simulink model "INS"  (R2018b)
settings: configuration reference "ins_config" (kept outside this file)
undefined symbols (not defined in the file): DiscIntNeverNeededParam, INS_CONST, INS_EXPORT, INS_EXPORT_VALUE, INS_PARAM, Sensor_Meas
libraries: simulink x155, FMT_Model_Lib x52
(part 5 of 6)

== system INS/Data_Fusion/Translation_Filter/TF_Data_PreProcess/Sensor_Process/TF_Sensor_Measures/ExternalPos_Meas/External_Pos_PreProcess ==
  Sensor_Data : Inport
  Rotation_Data : Inport  Port=2
  Bus Selector2 : BusSelector  OutputSignals=ExternalPos_Data.x,ExternalPos_Data.y,ExternalPos_Data.h
  Bus Selector5 : BusSelector  OutputSignals=ExternalPos_Data.timestamp
  Demux : Demux  Outputs=3
  Local_To_Global : Subsystem
  Multiply : Product  Multiplication=Matrix(*)
  Mux : Mux  Inputs=3
  Reshape : Reshape  OutputDimensionality=Column vector (2-D)
  timestamp : Outport  VectorParamsAs1DForOutWhenUnconnected=off
  x : Outport  Port=2  VectorParamsAs1DForOutWhenUnconnected=off
  y : Outport  Port=3  VectorParamsAs1DForOutWhenUnconnected=off
  h : Outport  Port=4  VectorParamsAs1DForOutWhenUnconnected=off
  wires:
  Bus Selector2/2 -> Mux/2  "<y>"
  Mux/1 -> Reshape/1  "xyh_local"
  Multiply/1 -> Demux/1
  Demux/1 -> x/1
  Demux/2 -> y/1
  Bus Selector2/3 -> Mux/3  "<h>"
  Reshape/1 -> Multiply/2
  Bus Selector2/1 -> Mux/1  "<x>"
  Demux/3 -> h/1
  Bus Selector5/1 -> timestamp/1  "<timestamp>"
  Sensor_Data/1 -> Bus Selector5/1, Local_To_Global/1(Sensor_Data), Bus Selector2/1
  Rotation_Data/1 -> Local_To_Global/2(Rotation_Data)
  Local_To_Global/1(M_OC) -> Multiply/1

== system INS/Data_Fusion/Translation_Filter/TF_Data_PreProcess/TF_Data_Post_Process/GPS_OFFSET_Compensation/GPS_POS_Compensation/WGS_To_Global ==
  TF_Data : Inport
  Bus Selector : BusSelector  OutputSignals=Sensor_Meas.GPS_Meas.lat_rad,Sensor_Meas.GPS_Meas.lon_rad,Sensor_Meas.GPS_Meas.h_m,TF_Control.WGS84_Ref.WGS84_pos_ref.lat_0_rad,TF_Control.WGS84_Ref.WGS84_pos_ref.lon_0_rad,TF_Control.WGS84_Ref.WGS84_pos_ref.h_0_m,TF_Control.WGS84_Ref.WGS84_derivatives_ref.dx_dlat_0,TF_Control.WGS84_Ref.WGS84_derivatives_ref.dy_dlon_0,TF_Control.WGS84_Ref.WGS84_derivatives_ref.dz_dh_0
  Multiply : Product
  Mux : Mux  Inputs=3
  Mux1 : Mux  Inputs=3
  Mux2 : Mux  Inputs=3
  Sum : Sum  Inputs=|+-
  pos_O_m : Outport  VectorParamsAs1DForOutWhenUnconnected=off
  wires:
  Bus Selector/2 -> Mux/2  "<lon_rad>"
  Bus Selector/6 -> Mux1/3  "<h_0_m>"
  Bus Selector/3 -> Mux/3  "<h_m>"
  Mux1/1 -> Sum/2
  Bus Selector/4 -> Mux1/1  "<lat_0_rad>"
  Sum/1 -> Multiply/1
  Mux2/1 -> Multiply/2
  Bus Selector/1 -> Mux/1  "<lat_rad>"
  Bus Selector/5 -> Mux1/2  "<lon_0_rad>"
  Mux/1 -> Sum/1
  TF_Data/1 -> Bus Selector/1
  Multiply/1 -> pos_O_m/1
  Bus Selector/7 -> Mux2/1  "<dx_dlat_0>"
  Bus Selector/8 -> Mux2/2  "<dy_dlon_0>"
  Bus Selector/9 -> Mux2/3  "<dz_dh_0>"

== system INS/Data_Fusion/Translation_Filter/TF_Data_PreProcess/TF_Data_Post_Process/GPS_OFFSET_Compensation/GPS_VEL_Compensation/delay ==
  u : Inport
  Divide : Product  Inputs=*/
  Mux : Mux  Inputs=3
  Selector : Selector  InputPortWidth=3  IndexOptions=Index vector (dialog)  Indices=1  OutputSizes=1
  Selector1 : Selector  InputPortWidth=3  IndexOptions=Index vector (dialog)  Indices=2  OutputSizes=1
  Selector2 : Selector  InputPortWidth=3  IndexOptions=Index vector (dialog)  Indices=3  OutputSizes=1
  gps_vd_delay : Delay  DelayLengthSource=Input port  DelayLength=INS_PARAM.GPS_VEL_DELAY/INS_EXPORT.period  DelayLengthUpperLimit=500  InitialConditionSource=Input port
      settings: InputPortMap=u0,p1,p4
  gps_ve_delay : Delay  DelayLengthSource=Input port  DelayLength=INS_PARAM.GPS_VEL_DELAY/INS_EXPORT.period  DelayLengthUpperLimit=500  InitialConditionSource=Input port
      settings: InputPortMap=u0,p1,p4
  gps_vnl_delay : Delay  DelayLengthSource=Input port  DelayLength=INS_PARAM.GPS_VEL_DELAY/INS_EXPORT.period  DelayLengthUpperLimit=500  InitialConditionSource=Input port
      settings: InputPortMap=u0,p1,p4
  period : Constant  Value=INS_EXPORT.period
  vel_delay : Constant  Value=INS_PARAM.GPS_VEL_DELAY
  y : Outport  VectorParamsAs1DForOutWhenUnconnected=off
  wires:
  u/1 -> Selector2/1, Selector1/1, Selector/1
  Divide/1 -> gps_vnl_delay/2, gps_vd_delay/2, gps_ve_delay/2
  vel_delay/1 -> Divide/1
  Selector/1 -> gps_vnl_delay/3, gps_vnl_delay/1
  Selector1/1 -> gps_ve_delay/3, gps_ve_delay/1
  Selector2/1 -> gps_vd_delay/3, gps_vd_delay/1
  gps_vnl_delay/1 -> Mux/1
  gps_ve_delay/1 -> Mux/2
  gps_vd_delay/1 -> Mux/3
  Mux/1 -> y/1
  period/1 -> Divide/2

== system INS/Data_Fusion/Translation_Filter/TF_Data_PreProcess/Transfer_Filter_Control/Sensor_Valid/Horizon_Sensor_Valid/valid_hold ==
  u : Inport
  Compare To Constant : simulink/Logic and Bit Operations/Compare To Constant  relop=>=  const=time_out  OutDataTypeStr=boolean
  Compare To Constant1 : simulink/Logic and Bit Operations/Compare To Constant  relop=>  const=0  OutDataTypeStr=boolean
  Compare To Constant2 : simulink/Logic and Bit Operations/Compare To Constant  relop=>  const=0  OutDataTypeStr=boolean
  Constant : Constant  Value=INS_EXPORT.period  OutDataTypeStr=uint32
  Delay : Delay  DelayLength=1
  Detect Rise Positive : simulink/Logic and Bit Operations/Detect Rise Positive  vinit=0  OutDataTypeStr=boolean
  Discrete-Time Integrator : DiscreteIntegrator  IntegratorMethod=Accumulation: Forward Euler  gainval=1  ExternalReset=level  SampleTime=-1  LimitOutput=on  UpperSaturationLimit=1e6  LowerSaturationLimit=0  ICPrevOutput=DiscIntNeverNeededParam  ICPrevScaledInput=DiscIntNeverNeededParam
  Logical Operator : Logic  Operator=NOT  AllPortsSameDT=off  OutDataTypeStr=boolean
  Logical Operator1 : Logic  Operator=OR  AllPortsSameDT=off  OutDataTypeStr=boolean
  Multiply : Product
  y : Outport  VectorParamsAs1DForOutWhenUnconnected=off
  wires:
  Multiply/1 -> y/1
  Logical Operator1/1 -> Multiply/2, Delay/1
  Detect Rise Positive/1 -> Logical Operator1/1
  Compare To Constant2/1 -> Detect Rise Positive/1
  u/1 -> Compare To Constant1/1, Compare To Constant2/1
  Compare To Constant1/1 -> Discrete-Time Integrator/2
  Constant/1 -> Discrete-Time Integrator/1
  Compare To Constant/1 -> Logical Operator/1
  Logical Operator/1 -> Multiply/1
  Discrete-Time Integrator/1 -> Compare To Constant/1
  Delay/1 -> Logical Operator1/2

== system INS/Data_Fusion/Translation_Filter/TF_Data_PreProcess/Transfer_Filter_Control/Sensor_Valid/Horizon_Sensor_Valid/valid_hold1 ==
  u : Inport
  Compare To Constant : simulink/Logic and Bit Operations/Compare To Constant  relop=>=  const=time_out  OutDataTypeStr=boolean
  Compare To Constant1 : simulink/Logic and Bit Operations/Compare To Constant  relop=>  const=0  OutDataTypeStr=boolean
  Compare To Constant2 : simulink/Logic and Bit Operations/Compare To Constant  relop=>  const=0  OutDataTypeStr=boolean
  Constant : Constant  Value=INS_EXPORT.period  OutDataTypeStr=uint32
  Delay : Delay  DelayLength=1
  Detect Rise Positive : simulink/Logic and Bit Operations/Detect Rise Positive  vinit=0  OutDataTypeStr=boolean
  Discrete-Time Integrator : DiscreteIntegrator  IntegratorMethod=Accumulation: Forward Euler  gainval=1  ExternalReset=level  SampleTime=-1  LimitOutput=on  UpperSaturationLimit=1e6  LowerSaturationLimit=0  ICPrevOutput=DiscIntNeverNeededParam  ICPrevScaledInput=DiscIntNeverNeededParam
  Logical Operator : Logic  Operator=NOT  AllPortsSameDT=off  OutDataTypeStr=boolean
  Logical Operator1 : Logic  Operator=OR  AllPortsSameDT=off  OutDataTypeStr=boolean
  Multiply : Product
  y : Outport  VectorParamsAs1DForOutWhenUnconnected=off
  wires:
  Discrete-Time Integrator/1 -> Compare To Constant/1
  Logical Operator/1 -> Multiply/1
  Compare To Constant/1 -> Logical Operator/1
  Constant/1 -> Discrete-Time Integrator/1
  Compare To Constant1/1 -> Discrete-Time Integrator/2
  u/1 -> Compare To Constant2/1, Compare To Constant1/1
  Compare To Constant2/1 -> Detect Rise Positive/1
  Detect Rise Positive/1 -> Logical Operator1/1
  Logical Operator1/1 -> Delay/1, Multiply/2
  Multiply/1 -> y/1
  Delay/1 -> Logical Operator1/2

== system INS/Data_Fusion/Translation_Filter/TF_Data_PreProcess/Transfer_Filter_Control/Sensor_Valid/Horizon_Sensor_Valid/valid_hold2 ==
  u : Inport
  Compare To Constant : simulink/Logic and Bit Operations/Compare To Constant  relop=>=  const=time_out  OutDataTypeStr=boolean
  Compare To Constant1 : simulink/Logic and Bit Operations/Compare To Constant  relop=>  const=0  OutDataTypeStr=boolean
  Compare To Constant2 : simulink/Logic and Bit Operations/Compare To Constant  relop=>  const=0  OutDataTypeStr=boolean
  Constant : Constant  Value=INS_EXPORT.period  OutDataTypeStr=uint32
  Delay : Delay  DelayLength=1
  Detect Rise Positive : simulink/Logic and Bit Operations/Detect Rise Positive  vinit=0  OutDataTypeStr=boolean
  Discrete-Time Integrator : DiscreteIntegrator  IntegratorMethod=Accumulation: Forward Euler  gainval=1  ExternalReset=level  SampleTime=-1  LimitOutput=on  UpperSaturationLimit=1e6  LowerSaturationLimit=0  ICPrevOutput=DiscIntNeverNeededParam  ICPrevScaledInput=DiscIntNeverNeededParam
  Logical Operator : Logic  Operator=NOT  AllPortsSameDT=off  OutDataTypeStr=boolean
  Logical Operator1 : Logic  Operator=OR  AllPortsSameDT=off  OutDataTypeStr=boolean
  Multiply : Product
  y : Outport  VectorParamsAs1DForOutWhenUnconnected=off
  wires:
  Delay/1 -> Logical Operator1/2
  Multiply/1 -> y/1
  Logical Operator1/1 -> Multiply/2, Delay/1
  Detect Rise Positive/1 -> Logical Operator1/1
  Compare To Constant2/1 -> Detect Rise Positive/1
  u/1 -> Compare To Constant1/1, Compare To Constant2/1
  Compare To Constant1/1 -> Discrete-Time Integrator/2
  Constant/1 -> Discrete-Time Integrator/1
  Compare To Constant/1 -> Logical Operator/1
  Logical Operator/1 -> Multiply/1
  Discrete-Time Integrator/1 -> Compare To Constant/1

== system INS/Data_Fusion/Translation_Filter/TF_Data_PreProcess/Transfer_Filter_Control/Sensor_Valid/Vertical_Sensor_Valid/valid_hold ==
  u : Inport
  Compare To Constant : simulink/Logic and Bit Operations/Compare To Constant  relop=>=  const=time_out  OutDataTypeStr=boolean
  Compare To Constant1 : simulink/Logic and Bit Operations/Compare To Constant  relop=>  const=0  OutDataTypeStr=boolean
  Compare To Constant2 : simulink/Logic and Bit Operations/Compare To Constant  relop=>  const=0  OutDataTypeStr=boolean
  Constant : Constant  Value=INS_EXPORT.period  OutDataTypeStr=uint32
  Delay : Delay  DelayLength=1
  Detect Rise Positive : simulink/Logic and Bit Operations/Detect Rise Positive  vinit=0  OutDataTypeStr=boolean
  Discrete-Time Integrator : DiscreteIntegrator  IntegratorMethod=Accumulation: Forward Euler  gainval=1  ExternalReset=level  SampleTime=-1  LimitOutput=on  UpperSaturationLimit=1e6  LowerSaturationLimit=0  ICPrevOutput=DiscIntNeverNeededParam  ICPrevScaledInput=DiscIntNeverNeededParam
  Logical Operator : Logic  Operator=NOT  AllPortsSameDT=off  OutDataTypeStr=boolean
  Logical Operator1 : Logic  Operator=OR  AllPortsSameDT=off  OutDataTypeStr=boolean
  Multiply : Product
  y : Outport  VectorParamsAs1DForOutWhenUnconnected=off
  wires:
  Multiply/1 -> y/1
  Logical Operator1/1 -> Multiply/2, Delay/1
  Detect Rise Positive/1 -> Logical Operator1/1
  Compare To Constant2/1 -> Detect Rise Positive/1
  u/1 -> Compare To Constant1/1, Compare To Constant2/1
  Compare To Constant1/1 -> Discrete-Time Integrator/2
  Constant/1 -> Discrete-Time Integrator/1
  Compare To Constant/1 -> Logical Operator/1
  Logical Operator/1 -> Multiply/1
  Discrete-Time Integrator/1 -> Compare To Constant/1
  Delay/1 -> Logical Operator1/2

== system INS/Data_Fusion/Translation_Filter/TF_Data_PreProcess/Transfer_Filter_Control/Sensor_Valid/Vertical_Sensor_Valid/valid_hold1 ==
  u : Inport
  Compare To Constant : simulink/Logic and Bit Operations/Compare To Constant  relop=>=  const=time_out  OutDataTypeStr=boolean
  Compare To Constant1 : simulink/Logic and Bit Operations/Compare To Constant  relop=>  const=0  OutDataTypeStr=boolean
  Compare To Constant2 : simulink/Logic and Bit Operations/Compare To Constant  relop=>  const=0  OutDataTypeStr=boolean
  Constant : Constant  Value=INS_EXPORT.period  OutDataTypeStr=uint32
  Delay : Delay  DelayLength=1
  Detect Rise Positive : simulink/Logic and Bit Operations/Detect Rise Positive  vinit=0  OutDataTypeStr=boolean
  Discrete-Time Integrator : DiscreteIntegrator  IntegratorMethod=Accumulation: Forward Euler  gainval=1  ExternalReset=level  SampleTime=-1  LimitOutput=on  UpperSaturationLimit=1e6  LowerSaturationLimit=0  ICPrevOutput=DiscIntNeverNeededParam  ICPrevScaledInput=DiscIntNeverNeededParam
  Logical Operator : Logic  Operator=NOT  AllPortsSameDT=off  OutDataTypeStr=boolean
  Logical Operator1 : Logic  Operator=OR  AllPortsSameDT=off  OutDataTypeStr=boolean
  Multiply : Product
  y : Outport  VectorParamsAs1DForOutWhenUnconnected=off
  wires:
  Discrete-Time Integrator/1 -> Compare To Constant/1
  Logical Operator/1 -> Multiply/1
  Compare To Constant/1 -> Logical Operator/1
  Constant/1 -> Discrete-Time Integrator/1
  Compare To Constant1/1 -> Discrete-Time Integrator/2
  u/1 -> Compare To Constant2/1, Compare To Constant1/1
  Compare To Constant2/1 -> Detect Rise Positive/1
  Detect Rise Positive/1 -> Logical Operator1/1
  Logical Operator1/1 -> Delay/1, Multiply/2
  Multiply/1 -> y/1
  Delay/1 -> Logical Operator1/2

== system INS/Data_Fusion/Translation_Filter/TF_Data_PreProcess/Transfer_Filter_Control/Sensor_Valid/Vertical_Sensor_Valid/valid_hold2 ==
  u : Inport
  Compare To Constant : simulink/Logic and Bit Operations/Compare To Constant  relop=>=  const=time_out  OutDataTypeStr=boolean
  Compare To Constant1 : simulink/Logic and Bit Operations/Compare To Constant  relop=>  const=0  OutDataTypeStr=boolean
  Compare To Constant2 : simulink/Logic and Bit Operations/Compare To Constant  relop=>  const=0  OutDataTypeStr=boolean
  Constant : Constant  Value=INS_EXPORT.period  OutDataTypeStr=uint32
  Delay : Delay  DelayLength=1
  Detect Rise Positive : simulink/Logic and Bit Operations/Detect Rise Positive  vinit=0  OutDataTypeStr=boolean
  Discrete-Time Integrator : DiscreteIntegrator  IntegratorMethod=Accumulation: Forward Euler  gainval=1  ExternalReset=level  SampleTime=-1  LimitOutput=on  UpperSaturationLimit=1e6  LowerSaturationLimit=0  ICPrevOutput=DiscIntNeverNeededParam  ICPrevScaledInput=DiscIntNeverNeededParam
  Logical Operator : Logic  Operator=NOT  AllPortsSameDT=off  OutDataTypeStr=boolean
  Logical Operator1 : Logic  Operator=OR  AllPortsSameDT=off  OutDataTypeStr=boolean
  Multiply : Product
  y : Outport  VectorParamsAs1DForOutWhenUnconnected=off
  wires:
  Delay/1 -> Logical Operator1/2
  Multiply/1 -> y/1
  Logical Operator1/1 -> Multiply/2, Delay/1
  Detect Rise Positive/1 -> Logical Operator1/1
  Compare To Constant2/1 -> Detect Rise Positive/1
  u/1 -> Compare To Constant1/1, Compare To Constant2/1
  Compare To Constant1/1 -> Discrete-Time Integrator/2
  Constant/1 -> Discrete-Time Integrator/1
  Compare To Constant/1 -> Logical Operator/1
  Logical Operator/1 -> Multiply/1
  Discrete-Time Integrator/1 -> Compare To Constant/1

== system INS/Data_Fusion/Rotation_Filter/AHRS/Correct/Attitude_Correction/Attitude_Correct/Acc_Correct/Heading_Correct ==
  acc_est_O_mPs2 : Inport
  acc_meas_O_mPs2 : Inport  Port=2
  acc_meas_valid : Inport  Port=3
  Cross Product : FMT_Model_Lib/Math/Cross Product
      settings: SourceProductName=FMT Toolbox
  Dead Zone2 : DeadZone  LowerValue=-0.2  UpperValue=0.2  SaturateOnIntegerOverflow=on
  Demux : Demux  Outputs=3
  Demux1 : Demux  Outputs=3
  Gain : Gain  Gain=INS_PARAM.HEADING_GAIN  OutDataTypeStr=single
  Gain1 : Gain  Gain=0
  Gain2 : Gain  Gain=0
  Multiply : Product
  Mux1 : Mux  Inputs=3
  Mux2 : Mux  Inputs=3
  Saturation : Saturate
  heading_correct : Outport  VectorParamsAs1DForOutWhenUnconnected=off
  wires:
  Dead Zone2/1 -> Gain/1
  Saturation/1 -> Multiply/1
  Mux1/1 -> Cross Product/2
  Cross Product/1 -> Dead Zone2/1
  Demux/1 -> Mux1/1
  acc_meas_valid/1 -> Multiply/2
  Multiply/1 -> heading_correct/1
  Gain/1 -> Saturation/1
  acc_meas_O_mPs2/1 -> Demux/1
  Demux/2 -> Mux1/2
  Demux/3 -> Gain1/1
  Gain1/1 -> Mux1/3
  Demux1/2 -> Mux2/2
  Mux2/1 -> Cross Product/1
  Gain2/1 -> Mux2/3
  Demux1/1 -> Mux2/1
  Demux1/3 -> Gain2/1
  acc_est_O_mPs2/1 -> Demux1/1

== system INS/Data_Fusion/Rotation_Filter/AHRS/Correct/Attitude_Correction/Attitude_Correct/Acc_Correct/Verticle_Correct ==
  acc_est_O_mPs2 : Inport
  acc_meas_O_mPs2 : Inport  Port=2
  Cross Product : FMT_Model_Lib/Math/Cross Product
      settings: SourceProductName=FMT Toolbox
  Demux : Demux  Outputs=3
  Gain : Gain  Gain=INS_PARAM.ATT_GAIN
  Gain1 : Gain  Gain=INS_PARAM.ATT_GAIN
  Gain2 : Gain  Gain=0
  Mux : Mux  Inputs=3
  Saturation : Subsystem
  Vector Normalize : FMT_Model_Lib/Math/Vector Normalize
      settings: SourceProductName=FMT Toolbox
  Vector Normalize1 : FMT_Model_Lib/Math/Vector Normalize
      settings: SourceProductName=FMT Toolbox
  vert_correct : Outport  VectorParamsAs1DForOutWhenUnconnected=off
  wires:
  Saturation/1(y) -> Demux/1
  Cross Product/1 -> Saturation/1(u)
  Vector Normalize/1 -> Cross Product/1
  acc_meas_O_mPs2/1 -> Vector Normalize1/1
  Mux/1 -> vert_correct/1
  acc_est_O_mPs2/1 -> Vector Normalize/1
  Vector Normalize1/1 -> Cross Product/2
  Demux/1 -> Gain/1
  Demux/2 -> Gain1/1
  Demux/3 -> Gain2/1
  Gain/1 -> Mux/1
  Gain1/1 -> Mux/2
  Gain2/1 -> Mux/3

== system INS/Data_Fusion/Rotation_Filter/AHRS/Correct/Attitude_Correction/Attitude_Correct/Acc_Estimator/Estimate_Acc ==
  gps_meas_valid : Inport
  Sensor_Data : Inport  Port=2
  Rotation_Data : Inport  Port=3
  Bus Selector : BusSelector  OutputSignals=IMU_Data.acc_B_mPs2
  Bus Selector1 : BusSelector  OutputSignals=M_OB
  Constant : Constant  Value=200  OutDataTypeStr=uint32
  Delay : Delay  DelayLengthSource=Input port  DelayLengthUpperLimit=200
      settings: InputPortMap=u0,p1
  Divide : Product  Inputs=*/
  GPS_Delay : Constant  Value=INS_EXPORT.period  OutDataTypeStr=uint32
  Multiply : Product  Multiplication=Matrix(*)
  Multiply2 : Product  OutDataTypeStr=single
  Second Order LPF : FMT_Model_Lib/Filter/Second Order LPF  fc=10  zeta=0.707
      settings: SourceProductName=FMT Toolbox
  acc_est_O_mPs2 : Outport  VectorParamsAs1DForOutWhenUnconnected=off
  wires:
  Second Order LPF/1 -> Delay/1
  Multiply/1 -> Second Order LPF/1  "acc_O"
  Bus Selector/1 -> Multiply/2  "<acc_B_mPs2>"
  Bus Selector1/1 -> Multiply/1  "<M_OB>"
  Rotation_Data/1 -> Bus Selector1/1
  Sensor_Data/1 -> Bus Selector/1
  Delay/1 -> acc_est_O_mPs2/1
  Multiply2/1 -> Delay/2
  Divide/1 -> Multiply2/2
  gps_meas_valid/1 -> Multiply2/1
  GPS_Delay/1 -> Divide/2
  Constant/1 -> Divide/1

== system INS/Data_Fusion/Rotation_Filter/AHRS/Correct/Attitude_Correction/Attitude_Correct/Acc_Estimator/Measure_Acc ==
  Sensor_Data : Inport
  Bus_Selection : Subsystem
  Detect Increase : simulink/Logic and Bit Operations/Detect Increase  vinit=0.0  OutDataTypeStr=boolean
  GPS_Meas_Acc : Subsystem  mask{fc=10, zeta=1}
      mask prompts: fc "Cut-off frequency (Hz)"; zeta "Damping factor"
  Valid_Check : Subsystem
  gps_meas_valid : Outport  VectorParamsAs1DForOutWhenUnconnected=off
  gps_meas_acc : Outport  Port=2  VectorParamsAs1DForOutWhenUnconnected=off
  wires:
  Valid_Check/1(gps_meas_acc_valid) -> gps_meas_valid/1, GPS_Meas_Acc/Enable, Detect Increase/1
  Detect Increase/1 -> GPS_Meas_Acc/1(reset)
  GPS_Meas_Acc/1(gps_acc_O_mPs2) -> gps_meas_acc/1
  Bus_Selection/1(gps_vel_O_mPs) -> GPS_Meas_Acc/2(gps_vel_O_mPs)
  Sensor_Data/1 -> Bus_Selection/1(Sensor_Data), Valid_Check/1(Sensor_Data)

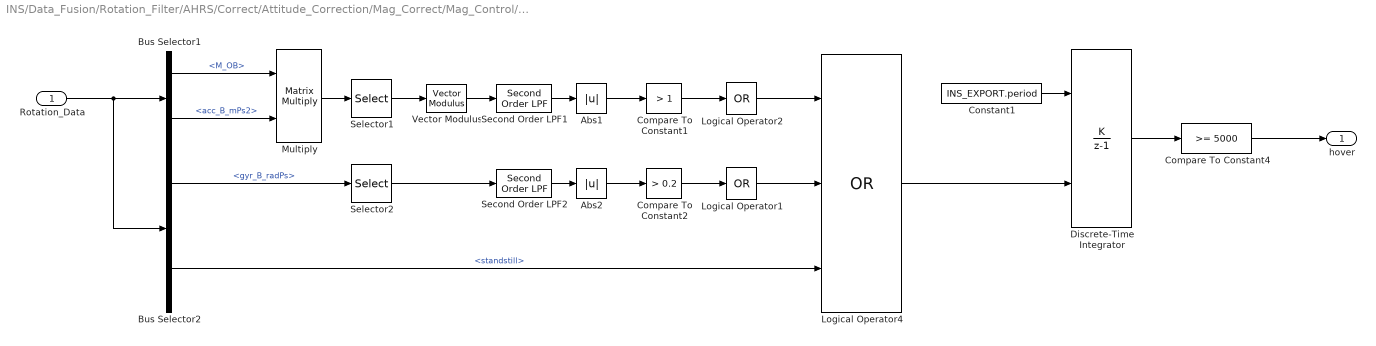
== system INS/Data_Fusion/Rotation_Filter/AHRS/Correct/Attitude_Correction/Mag_Correct/Mag_Control/Hover ==
  Rotation_Data : Inport
  Abs1 : Abs
  Abs2 : Abs
  Bus Selector1 : BusSelector  OutputSignals=M_OB,acc_B_mPs2
  Bus Selector2 : BusSelector  OutputSignals=gyr_B_radPs,standstill
  Compare To Constant1 : simulink/Logic and Bit Operations/Compare To Constant  relop=>  const=1  OutDataTypeStr=boolean
  Compare To Constant2 : simulink/Logic and Bit Operations/Compare To Constant  relop=>  const=0.2  OutDataTypeStr=boolean
  Compare To Constant4 : simulink/Logic and Bit Operations/Compare To Constant  relop=>=  const=5000  OutDataTypeStr=boolean
  Constant1 : Constant  Value=INS_EXPORT.period  OutDataTypeStr=uint32
  Discrete-Time Integrator : DiscreteIntegrator  IntegratorMethod=Accumulation: Forward Euler  ExternalReset=level  SampleTime=-1  OutDataTypeStr=uint32  SaturateOnIntegerOverflow=on  LimitOutput=on  UpperSaturationLimit=4294967295  LowerSaturationLimit=0  ICPrevOutput=DiscIntNeverNeededParam  ICPrevScaledInput=DiscIntNeverNeededParam
  Logical Operator1 : Logic  Operator=OR  Inputs=1  AllPortsSameDT=off  OutDataTypeStr=boolean
  Logical Operator2 : Logic  Operator=OR  Inputs=1  AllPortsSameDT=off  OutDataTypeStr=boolean
  Logical Operator4 : Logic  Operator=OR  Inputs=3  AllPortsSameDT=off  OutDataTypeStr=boolean
  Multiply : Product  Multiplication=Matrix(*)
  Second Order LPF1 : FMT_Model_Lib/Filter/Second Order LPF  fc=5  zeta=0.707
      settings: SourceProductName=FMT Toolbox
  Second Order LPF2 : FMT_Model_Lib/Filter/Second Order LPF  fc=5  zeta=0.707
      settings: SourceProductName=FMT Toolbox
  Selector1 : Selector  InputPortWidth=3  IndexOptions=Index vector (dialog)  Indices=[1 2]  OutputSizes=1
  Selector2 : Selector  InputPortWidth=3  IndexOptions=Index vector (dialog)  Indices=3  OutputSizes=1
  Vector Modulus : FMT_Model_Lib/Math/Vector Modulus
      settings: SourceProductName=FMT Toolbox
  hover : Outport  VectorParamsAs1DForOutWhenUnconnected=off
  wires:
  Discrete-Time Integrator/1 -> Compare To Constant4/1
  Logical Operator4/1 -> Discrete-Time Integrator/2
  Constant1/1 -> Discrete-Time Integrator/1
  Compare To Constant4/1 -> hover/1
  Rotation_Data/1 -> Bus Selector2/1, Bus Selector1/1
  Bus Selector1/2 -> Multiply/2  "<acc_B_mPs2>"
  Bus Selector1/1 -> Multiply/1  "<M_OB>"
  Multiply/1 -> Selector1/1
  Selector1/1 -> Vector Modulus/1
  Compare To Constant1/1 -> Logical Operator2/1
  Abs1/1 -> Compare To Constant1/1
  Logical Operator2/1 -> Logical Operator4/1
  Bus Selector2/1 -> Selector2/1  "<gyr_B_radPs>"
  Selector2/1 -> Second Order LPF2/1
  Second Order LPF2/1 -> Abs2/1
  Abs2/1 -> Compare To Constant2/1
  Compare To Constant2/1 -> Logical Operator1/1
  Logical Operator1/1 -> Logical Operator4/2
  Bus Selector2/2 -> Logical Operator4/3  "<standstill>"
  Second Order LPF1/1 -> Abs1/1
  Vector Modulus/1 -> Second Order LPF1/1

== system INS/Data_Fusion/Rotation_Filter/AHRS/Correct/Attitude_Correction/Mag_Correct/Mag_Measure/Bias_Estimation ==
  bias_update : Inport
  psi_meas : Inport  Port=2
  psi_est : Inport  Port=3
  standstill : Inport  Port=4
  Bias : Subsystem
  Delay : Delay  DelayLength=1
  Logical Operator1 : Logic  Operator=NOT  AllPortsSameDT=off  OutDataTypeStr=boolean
  Multiply : Product
  Switch : Switch  Criteria=u2 > Threshold  OutDataTypeStr=single
  bias : Outport  VectorParamsAs1DForOutWhenUnconnected=off
  wires:
  Delay/1 -> Switch/3
  Bias/1(bias) -> Switch/1
  Multiply/1 -> Delay/1, bias/1
  psi_meas/1 -> Bias/2(psi_meas)
  psi_est/1 -> Bias/1(psi_est)
  bias_update/1 -> Switch/2  "mag_bias_update"
  Switch/1 -> Multiply/2
  standstill/1 -> Logical Operator1/1
  Logical Operator1/1 -> Multiply/1

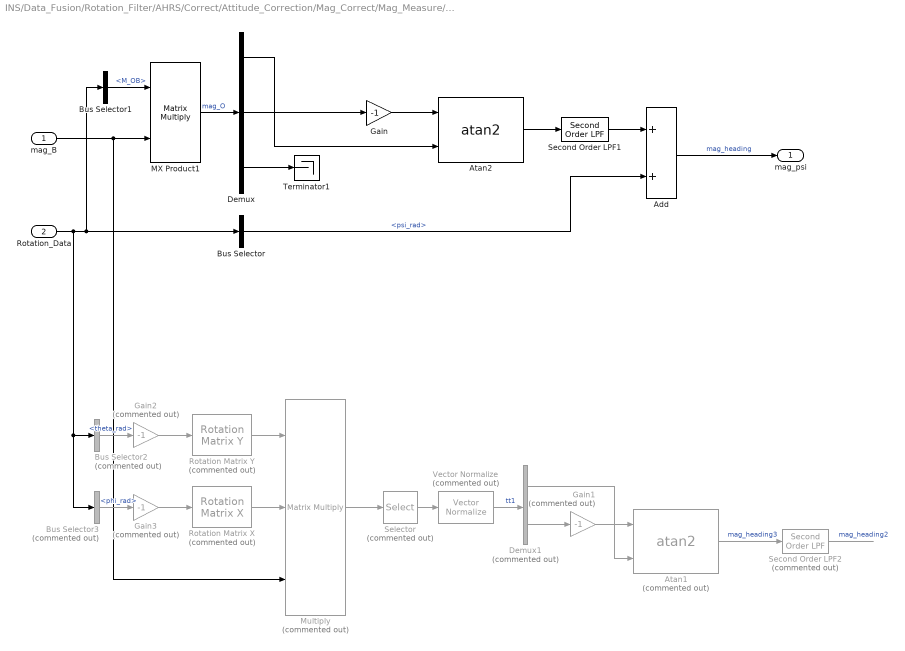
== system INS/Data_Fusion/Rotation_Filter/AHRS/Correct/Attitude_Correction/Mag_Correct/Mag_Measure/Mag_Heading ==
  mag_B : Inport
  Rotation_Data : Inport  Port=2
  Add : Sum
  Atan1 : Trigonometry  Commented=on  Operator=atan2
  Atan2 : Trigonometry  Operator=atan2
  Bus Selector : BusSelector  OutputSignals=psi_rad
  Bus Selector1 : BusSelector  OutputSignals=M_OB
  Bus Selector2 : BusSelector  Commented=on  OutputSignals=theta_rad
  Bus Selector3 : BusSelector  Commented=on  OutputSignals=phi_rad
  Demux : Demux  Outputs=3
  Demux1 : Demux  Commented=on  Outputs=2
  Gain : Gain  Gain=-1
  Gain1 : Gain  Commented=on  Gain=-1
  Gain2 : Gain  Commented=on  Gain=-1
  Gain3 : Gain  Commented=on  Gain=-1
  MX Product1 : Product  Multiplication=Matrix(*)  RndMeth=Simplest
  Multiply : Product  Commented=on  Inputs=3  Multiplication=Matrix(*)
  Rotation Matrix X : FMT_Model_Lib/Transformation/Rotation Matrix X  Commented=on
      settings: SourceProductName=FMT Toolbox
  Rotation Matrix Y : FMT_Model_Lib/Transformation/Rotation Matrix Y  Commented=on
      settings: SourceProductName=FMT Toolbox
  Second Order LPF1 : FMT_Model_Lib/Filter/Second Order LPF  fc=5  zeta=0.707
      settings: SourceProductName=FMT Toolbox
  Second Order LPF2 : FMT_Model_Lib/Filter/Second Order LPF  Commented=on  fc=5  zeta=0.707
      settings: SourceProductName=FMT Toolbox
  Selector : Selector  Commented=on  InputPortWidth=3  IndexOptions=Index vector (dialog)  Indices=[1 2]  OutputSizes=1
  Terminator1 : Terminator
  Vector Normalize : FMT_Model_Lib/Math/Vector Normalize  Commented=on
      settings: SourceProductName=FMT Toolbox
  mag_psi : Outport  VectorParamsAs1DForOutWhenUnconnected=off
  wires:
  Demux/3 -> Terminator1/1
  Atan2/1 -> Second Order LPF1/1
  Demux/1 -> Atan2/2
  MX Product1/1 -> Demux/1  "mag_O"
  Gain/1 -> Atan2/1
  Add/1 -> mag_psi/1  "mag_heading"
  Rotation_Data/1 -> Bus Selector3/1, Bus Selector2/1, Bus Selector1/1, Bus Selector/1
  Bus Selector/1 -> Add/2  "<psi_rad>"
  Demux/2 -> Gain/1
  mag_B/1 -> Multiply/3, MX Product1/2
  Bus Selector1/1 -> MX Product1/1  "<M_OB>"
  Second Order LPF1/1 -> Add/1
  Gain1/1 -> Atan1/1
  Atan1/1 -> Second Order LPF2/1  "mag_heading3"
  Second Order LPF2/1 -> ?  "mag_heading2"
  Selector/1 -> Vector Normalize/1
  Vector Normalize/1 -> Demux1/1  "tt1"
  Demux1/2 -> Gain1/1
  Demux1/1 -> Atan1/2
  Rotation Matrix Y/1 -> Multiply/1
  Rotation Matrix X/1 -> Multiply/2
  Bus Selector2/1 -> Gain2/1  "<theta_rad>"
  Gain3/1 -> Rotation Matrix X/1
  Gain2/1 -> Rotation Matrix Y/1
  Bus Selector3/1 -> Gain3/1  "<phi_rad>"
  Multiply/1 -> Selector/1

== system INS/Data_Fusion/Translation_Filter/CF/Bus_Constructor/Bus_Select/WGS84_Position/WGS84_Position/safe_divide ==
  u1 : Inport
  u2 : Inport  Port=2
  Divide : Product  Inputs=*/
  Zero_Value_Exclusion : Subsystem
  y : Outport  VectorParamsAs1DForOutWhenUnconnected=off
  wires:
  Zero_Value_Exclusion/1(y) -> Divide/2
  Divide/1 -> y/1
  u1/1 -> Divide/1
  u2/1 -> Zero_Value_Exclusion/1(u)

== system INS/Data_Fusion/Translation_Filter/CF/Horizontal_Filter/Correct/Airspeed Correct/Airspeed_Correct/Error_Integrate ==
  error : Inport
  update : Inport  Port=2
  Gain3 : Gain  Gain=INS_CONST.dt  OutDataTypeStr=Inherit: Same as input
  Memory : Memory
  Switch : Switch  Criteria=u2 > Threshold
  corr : Outport  VectorParamsAs1DForOutWhenUnconnected=off
  wires:
  Gain3/1 -> corr/1
  Memory/1 -> Switch/3
  error/1 -> Switch/1
  Switch/1 -> Gain3/1, Memory/1
  update/1 -> Switch/2

== system INS/Data_Fusion/Translation_Filter/CF/Horizontal_Filter/Correct/Airspeed Correct/Airspeed_Correct/Error_Scaling ==
  err_in : Inport
  Constant : Constant  Value=[0;0;0;0;0;0]  VectorParams1D=off  OutDataTypeStr=single
  Gain2 : Gain  Gain=2  OutDataTypeStr=single
  Mux : Mux  Inputs=2
  Reshape : Reshape  OutputDimensionality=Column vector (2-D)  OutputDimensions=[6,1]
  err_out : Outport  VectorParamsAs1DForOutWhenUnconnected=off
  wires:
  Reshape/1 -> err_out/1
  Mux/1 -> Reshape/1
  err_in/1 -> Gain2/1
  Gain2/1 -> Mux/2
  Constant/1 -> Mux/1

== system INS/Data_Fusion/Translation_Filter/CF/Horizontal_Filter/Correct/Airspeed Correct/Airspeed_Correct/Estimate_State ==
  X : Inport
  reset : Inport  Port=2
  Divide : Product  Inputs=*/
  IAS_delay : Constant  Value=10
  Selector : Selector  InputPortWidth=7  IndexOptions=Index vector (dialog)  Indices=7  OutputSizes=1
  airspeed_delay : Delay  DelayLengthSource=Input port  DelayLength=INS_PARAM.EXTPOS_POS_DELAY/INS_EXPORT.period  DelayLengthUpperLimit=500  InitialConditionSource=Input port  ExternalReset=Rising
      settings: InputPortMap=u0,p1,r5,p4
  period : Constant  Value=INS_EXPORT.period
  HX : Outport  VectorParamsAs1DForOutWhenUnconnected=off
  wires:
  Divide/1 -> airspeed_delay/2
  IAS_delay/1 -> Divide/1
  X/1 -> Selector/1
  Selector/1 -> airspeed_delay/4, airspeed_delay/1
  airspeed_delay/1 -> HX/1
  reset/1 -> airspeed_delay/3
  period/1 -> Divide/2

== system INS/Data_Fusion/Translation_Filter/CF/Horizontal_Filter/Correct/Airspeed Correct/Airspeed_Correct/Measurement ==
  TF_Data : Inport
  Bus Selector : BusSelector  OutputSignals=Sensor_Meas.Airspeed_Meas.IAS_mPs
  Z : Outport  VectorParamsAs1DForOutWhenUnconnected=off
  wires:
  Bus Selector/1 -> Z/1  "<IAS_mPs>"
  TF_Data/1 -> Bus Selector/1

== system INS/Data_Fusion/Translation_Filter/CF/Horizontal_Filter/Correct/ExternalPos Correct/ExternalPos_Correct/Error_Integrate ==
  error : Inport
  update : Inport  Port=2
  Gain3 : Gain  Gain=INS_CONST.dt  OutDataTypeStr=Inherit: Same as input
  Memory : Memory
  Switch : Switch  Criteria=u2 > Threshold
  corr : Outport  VectorParamsAs1DForOutWhenUnconnected=off
  wires:
  update/1 -> Switch/2
  Switch/1 -> Memory/1, Gain3/1
  error/1 -> Switch/1
  Memory/1 -> Switch/3
  Gain3/1 -> corr/1

== system INS/Data_Fusion/Translation_Filter/CF/Horizontal_Filter/Correct/ExternalPos Correct/ExternalPos_Correct/Error_Scaling ==
  err_in : Inport
  Constant1 : Constant  Value=0  VectorParams1D=off  OutDataTypeStr=single
  Gain : Gain  Gain=INS_PARAM.EXTPOS_VEL_GAIN  OutDataTypeStr=single
  Gain2 : Gain  Gain=-INS_PARAM.EXTPOS_BIAS_A_GAIN  OutDataTypeStr=single
  Gain3 : Gain  Gain=INS_PARAM.EXTPOS_POS_GAIN  OutDataTypeStr=single
  Mux : Mux
  Reshape : Reshape  OutputDimensionality=Column vector (2-D)  OutputDimensions=[6,1]
  err_out : Outport  VectorParamsAs1DForOutWhenUnconnected=off
  wires:
  err_in/1 -> Gain3/1, Gain2/1, Gain/1
  Gain2/1 -> Mux/3
  Mux/1 -> Reshape/1
  Gain3/1 -> Mux/1
  Gain/1 -> Mux/2
  Reshape/1 -> err_out/1
  Constant1/1 -> Mux/4

== system INS/Data_Fusion/Translation_Filter/CF/Horizontal_Filter/Correct/ExternalPos Correct/ExternalPos_Correct/Estimate_State ==
  X : Inport
  reset : Inport  Port=2
  Divide : Product  Inputs=*/
  Mux : Mux  Inputs=2
  Reshape : Reshape  OutputDimensionality=Column vector (2-D)  OutputDimensions=[4,1]
  Selector : Selector  InputPortWidth=7  IndexOptions=Index vector (dialog)  Indices=[1]  OutputSizes=1
  Selector1 : Selector  InputPortWidth=7  IndexOptions=Index vector (dialog)  Indices=[2]  OutputSizes=1
  period : Constant  Value=INS_EXPORT.period
  pos_delay : Constant  Value=INS_PARAM.EXTPOS_POS_DELAY
  x_delay : Delay  DelayLengthSource=Input port  DelayLength=INS_PARAM.EXTPOS_POS_DELAY/INS_EXPORT.period  DelayLengthUpperLimit=500  InitialConditionSource=Input port  ExternalReset=Rising
      settings: InputPortMap=u0,p1,r5,p4
  y_delay : Delay  DelayLengthSource=Input port  DelayLength=INS_PARAM.EXTPOS_POS_DELAY/INS_EXPORT.period  DelayLengthUpperLimit=500  InitialConditionSource=Input port  ExternalReset=Rising
      settings: InputPortMap=u0,p1,r5,p4
  HX : Outport  VectorParamsAs1DForOutWhenUnconnected=off
  wires:
  Mux/1 -> Reshape/1
  Reshape/1 -> HX/1
  reset/1 -> x_delay/3, y_delay/3
  y_delay/1 -> Mux/2
  x_delay/1 -> Mux/1
  Selector/1 -> x_delay/1, x_delay/4
  X/1 -> Selector1/1, Selector/1
  Selector1/1 -> y_delay/4, y_delay/1
  pos_delay/1 -> Divide/1
  Divide/1 -> y_delay/2, x_delay/2
  period/1 -> Divide/2

== system INS/Data_Fusion/Translation_Filter/CF/Horizontal_Filter/Correct/ExternalPos Correct/ExternalPos_Correct/Measurement ==
  X : Inport
  TF_Data : Inport  Port=2
  Bias_Estimation : Subsystem
  Bus Selector : BusSelector  OutputSignals=Sensor_Meas.ExtPos_Meas.x_O_m,Sensor_Meas.ExtPos_Meas.y_O_m
  Mux : Mux  Inputs=2
  Sum1 : Sum  Inputs=|++
  Z : Outport  VectorParamsAs1DForOutWhenUnconnected=off
  bias_update : Outport  Port=2  VectorParamsAs1DForOutWhenUnconnected=off
  wires:
  Bias_Estimation/1(bias) -> Sum1/2
  X/1 -> Bias_Estimation/3(X)
  TF_Data/1 -> Bias_Estimation/2(TF_Data), Bus Selector/1
  Sum1/1 -> Z/1
  Bias_Estimation/2(bias_update) -> bias_update/1
  Mux/1 -> Bias_Estimation/1(meas), Sum1/1
  Bus Selector/1 -> Mux/1  "<x_O_m>"
  Bus Selector/2 -> Mux/2  "<y_O_m>"

== system INS/Data_Fusion/Translation_Filter/CF/Horizontal_Filter/Correct/GPS Correct/GPS_Correct/Error_Integrate ==
  error : Inport
  update : Inport  Port=2
  Gain3 : Gain  Gain=INS_CONST.dt  OutDataTypeStr=Inherit: Same as input
  Memory : Memory
  Switch : Switch  Criteria=u2 > Threshold
  corr : Outport  VectorParamsAs1DForOutWhenUnconnected=off
  wires:
  update/1 -> Switch/2
  Switch/1 -> Memory/1, Gain3/1
  error/1 -> Switch/1
  Memory/1 -> Switch/3
  Gain3/1 -> corr/1

== system INS/Data_Fusion/Translation_Filter/CF/Horizontal_Filter/Correct/GPS Correct/GPS_Correct/Error_Scaling ==
  err_in : Inport
  rtk_valid : Inport  Port=2
  GPS_Error_Scaling : Subsystem
  RTK_Error_Scaling : Subsystem
  Reshape : Reshape  OutputDimensionality=Column vector (2-D)  OutputDimensions=[7,1]
  Switch : Switch  Criteria=u2 > Threshold
  err_out : Outport  VectorParamsAs1DForOutWhenUnconnected=off
  wires:
  Reshape/1 -> err_out/1
  err_in/1 -> RTK_Error_Scaling/1(err_in), GPS_Error_Scaling/1(err_in)
  Switch/1 -> Reshape/1
  GPS_Error_Scaling/1(err_out) -> Switch/3
  RTK_Error_Scaling/1(err_out) -> Switch/1
  rtk_valid/1 -> Switch/2

== system INS/Data_Fusion/Translation_Filter/CF/Horizontal_Filter/Correct/GPS Correct/GPS_Correct/Estimate_State ==
  X : Inport
  reset : Inport  Port=2
  Divide : Product  Inputs=*/
  Divide1 : Product  Inputs=*/
  Mux : Mux
  Reshape : Reshape  OutputDimensionality=Customize  OutputDimensions=[4,1]
  Selector : Selector  InputPortWidth=7  IndexOptions=Index vector (dialog)  Indices=[1]  OutputSizes=1
  Selector1 : Selector  InputPortWidth=7  IndexOptions=Index vector (dialog)  Indices=[2]  OutputSizes=1
  Selector2 : Selector  InputPortWidth=7  IndexOptions=Index vector (dialog)  Indices=[3]  OutputSizes=1
  Selector3 : Selector  InputPortWidth=7  IndexOptions=Index vector (dialog)  Indices=[4]  OutputSizes=1
  period : Constant  Value=INS_EXPORT.period
  pos_delay : Constant  Value=INS_PARAM.GPS_POS_DELAY
  ve_delay : Delay  DelayLengthSource=Input port  DelayLength=INS_PARAM.GPS_VEL_DELAY/INS_EXPORT.period  DelayLengthUpperLimit=500  InitialConditionSource=Input port  ExternalReset=Rising
      settings: InputPortMap=u0,p1,r5,p4
  vel_delay : Constant  Value=INS_PARAM.GPS_VEL_DELAY
  vn_delay : Delay  DelayLengthSource=Input port  DelayLength=INS_PARAM.GPS_VEL_DELAY/INS_EXPORT.period  DelayLengthUpperLimit=500  InitialConditionSource=Input port  ExternalReset=Rising
      settings: InputPortMap=u0,p1,r5,p4
  x_delay : Delay  DelayLengthSource=Input port  DelayLength=INS_PARAM.GPS_POS_DELAY/INS_EXPORT.period  DelayLengthUpperLimit=500  InitialConditionSource=Input port  ExternalReset=Rising
      settings: InputPortMap=u0,p1,r5,p4
  y_delay : Delay  DelayLengthSource=Input port  DelayLength=INS_PARAM.GPS_POS_DELAY/INS_EXPORT.period  InitialConditionSource=Input port  ExternalReset=Rising
      settings: InputPortMap=u0,p1,r5,p4
  HX : Outport  VectorParamsAs1DForOutWhenUnconnected=off
  wires:
  Mux/1 -> Reshape/1
  Reshape/1 -> HX/1
  reset/1 -> x_delay/3, y_delay/3, vn_delay/3, ve_delay/3
  y_delay/1 -> Mux/2
  vn_delay/1 -> Mux/3
  ve_delay/1 -> Mux/4
  x_delay/1 -> Mux/1
  Selector/1 -> x_delay/1, x_delay/4
  X/1 -> Selector3/1, Selector2/1, Selector1/1, Selector/1
  Selector1/1 -> y_delay/4, y_delay/1
  Selector2/1 -> vn_delay/1, vn_delay/4
  Selector3/1 -> ve_delay/1, ve_delay/4
  pos_delay/1 -> Divide/1
  Divide/1 -> y_delay/2, x_delay/2
  vel_delay/1 -> Divide1/1
  Divide1/1 -> ve_delay/2, vn_delay/2
  period/1 -> Divide/2, Divide1/2

== system INS/Data_Fusion/Translation_Filter/CF/Horizontal_Filter/Correct/GPS Correct/GPS_Correct/Measurement ==
  X : Inport
  TF_Data : Inport  Port=2
  Bias_Estimation : Subsystem
  Bus Selector1 : BusSelector  OutputSignals=Sensor_Meas.GPS_Meas.vn_mPs,Sensor_Meas.GPS_Meas.ve_mPs
  Bus Selector2 : BusSelector  OutputSignals=Sensor_Meas.GPS_Meas.x_m,Sensor_Meas.GPS_Meas.y_m
  Data Type Conversion : DataTypeConversion  OutDataTypeStr=single
  Mux3 : Mux  Inputs=2
  Mux4 : Mux  Inputs=2
  Mux5 : Mux  Inputs=2
  Reshape3 : Reshape  OutputDimensionality=Customize  OutputDimensions=[4,1]
  Z : Outport  VectorParamsAs1DForOutWhenUnconnected=off
  bias_update : Outport  Port=2  VectorParamsAs1DForOutWhenUnconnected=off
  wires:
  X/1 -> Bias_Estimation/2(X)
  Data Type Conversion/1 -> Bias_Estimation/3(xy_meas_m)
  Bias_Estimation/2(xy_O_m) -> Mux3/1
  Bus Selector1/2 -> Mux4/2  "<ve_mPs>"
  Bus Selector1/1 -> Mux4/1  "<vn_mPs>"
  TF_Data/1 -> Bus Selector1/1, Bus Selector2/1, Bias_Estimation/1(TF_Data)
  Bias_Estimation/1(bias_update) -> bias_update/1
  Mux3/1 -> Reshape3/1
  Reshape3/1 -> Z/1
  Mux4/1 -> Mux3/2
  Bus Selector2/1 -> Mux5/1  "<x_m>"
  Bus Selector2/2 -> Mux5/2  "<y_m>"
  Mux5/1 -> Data Type Conversion/1

== system INS/Data_Fusion/Translation_Filter/CF/Horizontal_Filter/Correct/OptFlow Correct/OptFlow_Correct/Error_Integrate ==
  error : Inport
  update : Inport  Port=2
  Gain3 : Gain  Gain=INS_CONST.dt  OutDataTypeStr=Inherit: Same as input
  Memory : Memory
  Switch : Switch  Criteria=u2 > Threshold
  corr : Outport  VectorParamsAs1DForOutWhenUnconnected=off
  wires:
  update/1 -> Switch/2
  Switch/1 -> Memory/1, Gain3/1
  error/1 -> Switch/1
  Memory/1 -> Switch/3
  Gain3/1 -> corr/1

== system INS/Data_Fusion/Translation_Filter/CF/Horizontal_Filter/Correct/OptFlow Correct/OptFlow_Correct/Error_Scaling ==
  err_in : Inport
  Constant : Constant  Value=[0;0]  VectorParams1D=off  OutDataTypeStr=single
  Constant1 : Constant  Value=0  VectorParams1D=off  OutDataTypeStr=single
  Gain : Gain  Gain=INS_PARAM.OPF_VEL_GAIN  OutDataTypeStr=single
  Gain2 : Gain  Gain=-INS_PARAM.OPF_BIAS_A_GAIN  OutDataTypeStr=single
  Mux : Mux
  Reshape : Reshape  OutputDimensionality=Column vector (2-D)  OutputDimensions=[6,1]
  err_out : Outport  VectorParamsAs1DForOutWhenUnconnected=off
  wires:
  err_in/1 -> Gain2/1, Gain/1
  Gain2/1 -> Mux/3
  Mux/1 -> Reshape/1
  Constant/1 -> Mux/1
  Gain/1 -> Mux/2
  Reshape/1 -> err_out/1
  Constant1/1 -> Mux/4

== system INS/Data_Fusion/Translation_Filter/CF/Horizontal_Filter/Correct/OptFlow Correct/OptFlow_Correct/Estimate_State ==
  X : Inport
  reset : Inport  Port=2
  Delay : Constant  Value=INS_PARAM.OPF_VEL_DELAY
  Divide : Product  Inputs=*/
  Mux : Mux  Inputs=2
  Reshape : Reshape  OutputDimensionality=Column vector (2-D)  OutputDimensions=[2,1]
  Selector2 : Selector  InputPortWidth=7  IndexOptions=Index vector (dialog)  Indices=[3]  OutputSizes=1
  Selector3 : Selector  InputPortWidth=7  IndexOptions=Index vector (dialog)  Indices=[4]  OutputSizes=1
  period : Constant  Value=INS_EXPORT.period
  ve_delay : Delay  DelayLengthSource=Input port  DelayLength=INS_PARAM.OPF_VEL_DELAY/INS_EXPORT.period  DelayLengthUpperLimit=500  InitialConditionSource=Input port  ExternalReset=Rising
      settings: InputPortMap=u0,p1,r5,p4
  vn_delay : Delay  DelayLengthSource=Input port  DelayLength=INS_PARAM.OPF_VEL_DELAY/INS_EXPORT.period  DelayLengthUpperLimit=500  InitialConditionSource=Input port  ExternalReset=Rising
      settings: InputPortMap=u0,p1,r5,p4
  HX : Outport  VectorParamsAs1DForOutWhenUnconnected=off
  wires:
  Mux/1 -> Reshape/1
  Reshape/1 -> HX/1
  reset/1 -> vn_delay/3, ve_delay/3
  X/1 -> Selector3/1, Selector2/1
  Selector2/1 -> vn_delay/4, vn_delay/1
  Selector3/1 -> ve_delay/1, ve_delay/4
  vn_delay/1 -> Mux/1
  ve_delay/1 -> Mux/2
  Delay/1 -> Divide/1
  Divide/1 -> ve_delay/2, vn_delay/2
  period/1 -> Divide/2

== system INS/Data_Fusion/Translation_Filter/CF/Horizontal_Filter/Correct/OptFlow Correct/OptFlow_Correct/Measurement ==
  TF_Data : Inport
  Bus Selector1 : BusSelector  OutputSignals=Sensor_Meas.OptFlow_Meas.vx_O_mPs,Sensor_Meas.OptFlow_Meas.vy_O_mPs
  Mux4 : Mux  Inputs=2
  Reshape3 : Reshape  OutputDimensionality=Column vector (2-D)  OutputDimensions=[2,1]
  Z : Outport  VectorParamsAs1DForOutWhenUnconnected=off
  wires:
  Bus Selector1/2 -> Mux4/2  "<vy_O_mPs>"
  Bus Selector1/1 -> Mux4/1  "<vx_O_mPs>"
  TF_Data/1 -> Bus Selector1/1
  Mux4/1 -> Reshape3/1
  Reshape3/1 -> Z/1

== system INS/Data_Fusion/Translation_Filter/CF/Horizontal_Filter/Predict/Propagate/States_Init/Pos_Init ==
  TF_Data : Inport
  Bus Selector : BusSelector  OutputSignals=Sensor_Enable.horizon_select.gps_enable
  Bus Selector1 : BusSelector  OutputSignals=Sensor_Enable.horizon_select.extpos_enable
  External_Pos_Init : Subsystem
  GPS_Pos_Init : Subsystem
  Merge : Merge
  XY_0 : Outport  VectorParamsAs1DForOutWhenUnconnected=off
  wires:
  TF_Data/1 -> Bus Selector1/1, External_Pos_Init/1(TF_Data), GPS_Pos_Init/1(TF_Data), Bus Selector/1
  GPS_Pos_Init/1(XY_0) -> Merge/1  "xy_0"
  Bus Selector/1 -> GPS_Pos_Init/Enable  "<gps_enable>"
  Bus Selector1/1 -> External_Pos_Init/Enable  "<extpos_enable>"
  External_Pos_Init/1(XY_0) -> Merge/2  "xy_0"
  Merge/1 -> XY_0/1

== system INS/Data_Fusion/Translation_Filter/CF/Horizontal_Filter/Predict/Propagate/States_Init/Vel_Init ==
  TF_Data : Inport
  Bus Selector : BusSelector  OutputSignals=Sensor_Enable.horizon_select.gps_enable
  Bus Selector1 : BusSelector  OutputSignals=Sensor_Enable.horizon_select.optflow_enable
  GPS_Vel_Init : Subsystem
  Merge : Merge
  OptFlow_Vel_Init : Subsystem
  vel_NE_0 : Outport  VectorParamsAs1DForOutWhenUnconnected=off
  wires:
  Bus Selector/1 -> GPS_Vel_Init/Enable  "<gps_enable>"
  TF_Data/1 -> Bus Selector1/1, OptFlow_Vel_Init/1(Processed_Data), GPS_Vel_Init/1(Processed_Data), Bus Selector/1
  Bus Selector1/1 -> OptFlow_Vel_Init/Enable  "<optflow_enable>"
  GPS_Vel_Init/1(Vel_NE_0) -> Merge/1
  OptFlow_Vel_Init/1(Vel_NE_0) -> Merge/2
  Merge/1 -> vel_NE_0/1

== system INS/Data_Fusion/Translation_Filter/CF/Verticle_Filter/Correct/Baro_Correct/Baro_Correct/Error_Hold ==
  in : Inport
  update : Inport  Port=2
  Delay : Delay  DelayLength=1
  Gain : Gain  Gain=INS_CONST.dt  OutDataTypeStr=Inherit: Same as input
  Switch : Switch  Criteria=u2 > Threshold
  out : Outport  VectorParamsAs1DForOutWhenUnconnected=off
  wires:
  update/1 -> Switch/2
  Switch/1 -> Delay/1, Gain/1
  in/1 -> Switch/1
  Delay/1 -> Switch/3
  Gain/1 -> out/1

== system INS/Data_Fusion/Translation_Filter/CF/Verticle_Filter/Correct/Baro_Correct/Baro_Correct/Error_Scaling ==
  errror_in : Inport
  Gain : Gain  Gain=INS_PARAM.BARO_BIAS_AZ_GAIN
  Gain1 : Gain  Gain=-INS_PARAM.BARO_VZ_GAIN
  Gain2 : Gain  Gain=INS_PARAM.BARO_H_GAIN
  Mux : Mux  Inputs=3
  Saturation : Saturate  UpperLimit=1  LowerLimit=-1
  errror_out : Outport  VectorParamsAs1DForOutWhenUnconnected=off
  wires:
  errror_in/1 -> Saturation/1
  Gain2/1 -> Mux/1
  Gain1/1 -> Mux/2
  Gain/1 -> Mux/3
  Mux/1 -> errror_out/1
  Saturation/1 -> Gain/1, Gain2/1, Gain1/1

== system INS/Data_Fusion/Translation_Filter/CF/Verticle_Filter/Correct/Baro_Correct/Baro_Correct/Estimate_States ==
  note: Delay compensate due to sensor
      | measurement delay
  X : Inport
  reset : Inport  Port=2
  Divide : Product  Inputs=*/
  Selector : Selector  InputPortWidth=3  IndexOptions=Index vector (dialog)  Indices=[1]  OutputSizes=1
  delay : Constant  Value=INS_PARAM.BARO_H_DELAY
  period : Constant  Value=INS_EXPORT.period
  x_delay : Delay  DelayLengthSource=Input port  DelayLength=INS_PARAM.BARO_H_DELAY/INS_EXPORT_VALUE.period  DelayLengthUpperLimit=500  InitialConditionSource=Input port  ExternalReset=Rising
      settings: InputPortMap=u0,p1,r5,p4
  HX : Outport  VectorParamsAs1DForOutWhenUnconnected=off
  wires:
  reset/1 -> x_delay/3
  Selector/1 -> x_delay/4, x_delay/1  "HX"
  X/1 -> Selector/1
  x_delay/1 -> HX/1
  Divide/1 -> x_delay/2
  delay/1 -> Divide/1
  period/1 -> Divide/2

== system INS/Data_Fusion/Translation_Filter/CF/Verticle_Filter/Correct/Baro_Correct/Baro_Correct/Measurement ==
  X : Inport
  TF_Data : Inport  Port=2
  Bias_Estimation : Subsystem
  Bus Selector : BusSelector  OutputSignals=Sensor_Meas.Baro_Meas.h_R_m
  Bus Selector1 : BusSelector  OutputSignals=Sensor_Meas.Baro_Meas.h_R_filter_m
  Sum1 : Sum  Inputs=|++
  Z : Outport  VectorParamsAs1DForOutWhenUnconnected=off
  bias_update : Outport  Port=2  VectorParamsAs1DForOutWhenUnconnected=off
  wires:
  Bus Selector/1 -> Sum1/1  "<h_R_m>"
  Bias_Estimation/1(bias) -> Sum1/2
  X/1 -> Bias_Estimation/3(X)
  TF_Data/1 -> Bias_Estimation/2(TF_Data), Bus Selector1/1, Bus Selector/1
  Sum1/1 -> Z/1
  Bias_Estimation/2(bias_update) -> bias_update/1
  Bus Selector1/1 -> Bias_Estimation/1(h_m)  "<h_R_filter_m>"

== system INS/Data_Fusion/Translation_Filter/CF/Verticle_Filter/Correct/ExternalPos_Correct/ExternalPos_Correct/Error_Hold ==
  in : Inport
  update : Inport  Port=2
  Delay : Delay  DelayLength=1
  Gain : Gain  Gain=INS_CONST.dt  OutDataTypeStr=Inherit: Same as input
  Switch : Switch  Criteria=u2 > Threshold
  out : Outport  VectorParamsAs1DForOutWhenUnconnected=off
  wires:
  update/1 -> Switch/2
  Switch/1 -> Delay/1, Gain/1
  in/1 -> Switch/1
  Delay/1 -> Switch/3
  Gain/1 -> out/1

== system INS/Data_Fusion/Translation_Filter/CF/Verticle_Filter/Correct/ExternalPos_Correct/ExternalPos_Correct/Error_Scaling ==
  errror_in : Inport
  Gain : Gain  Gain=INS_PARAM.EXTPOS_BIAS_A_GAIN
  Gain1 : Gain  Gain=-INS_PARAM.EXTPOS_VEL_GAIN
  Gain2 : Gain  Gain=INS_PARAM.EXTPOS_POS_GAIN
  Mux : Mux  Inputs=3
  Saturation : Saturate  UpperLimit=1  LowerLimit=-1
  errror_out : Outport  VectorParamsAs1DForOutWhenUnconnected=off
  wires:
  errror_in/1 -> Saturation/1
  Gain2/1 -> Mux/1
  Gain1/1 -> Mux/2
  Gain/1 -> Mux/3
  Mux/1 -> errror_out/1
  Saturation/1 -> Gain/1, Gain2/1, Gain1/1

== system INS/Data_Fusion/Translation_Filter/CF/Verticle_Filter/Correct/ExternalPos_Correct/ExternalPos_Correct/Estimate_States ==
  note: Delay compensate due to sensor
      | measurement delay
  X : Inport
  reset : Inport  Port=2
  Divide : Product  Inputs=*/
  Selector : Selector  InputPortWidth=3  IndexOptions=Index vector (dialog)  Indices=[1]  OutputSizes=1
  delay : Constant  Value=INS_PARAM.EXTPOS_POS_DELAY
  period : Constant  Value=INS_EXPORT.period
  x_delay : Delay  DelayLengthSource=Input port  DelayLength=INS_PARAM.EXTPOS_POS_DELAY/INS_EXPORT_VALUE.period  DelayLengthUpperLimit=500  InitialConditionSource=Input port  ExternalReset=Rising
      settings: InputPortMap=u0,p1,r5,p4
  HX : Outport  VectorParamsAs1DForOutWhenUnconnected=off
  wires:
  reset/1 -> x_delay/3
  Selector/1 -> x_delay/4, x_delay/1  "HX"
  X/1 -> Selector/1
  x_delay/1 -> HX/1
  Divide/1 -> x_delay/2
  delay/1 -> Divide/1
  period/1 -> Divide/2

== system INS/Data_Fusion/Translation_Filter/CF/Verticle_Filter/Correct/ExternalPos_Correct/ExternalPos_Correct/Measurement ==
  X : Inport
  TF_Data : Inport  Port=2
  Bias_Estimation : Subsystem
  Bus Selector : BusSelector  OutputSignals=Sensor_Meas.ExtPos_Meas.h_O_m
  Sum1 : Sum  Inputs=|++
  Z : Outport  VectorParamsAs1DForOutWhenUnconnected=off
  bias_update : Outport  Port=2  VectorParamsAs1DForOutWhenUnconnected=off
  wires:
  Bus Selector/1 -> Bias_Estimation/1(h_m), Sum1/1  "<h_O_m>"
  Bias_Estimation/1(bias) -> Sum1/2
  X/1 -> Bias_Estimation/3(X)
  TF_Data/1 -> Bias_Estimation/2(TF_Data), Bus Selector/1
  Sum1/1 -> Z/1
  Bias_Estimation/2(bias_update) -> bias_update/1

== system INS/Data_Fusion/Translation_Filter/CF/Verticle_Filter/Correct/GPS_Correct/GPS_Correct/Error_Hold ==
  in : Inport
  update : Inport  Port=2
  Gain3 : Gain  Gain=INS_CONST.dt  OutDataTypeStr=Inherit: Same as input
  Memory : Memory
  Switch : Switch  Criteria=u2 > Threshold
  out : Outport  VectorParamsAs1DForOutWhenUnconnected=off
  wires:
  update/1 -> Switch/2
  Switch/1 -> Memory/1, Gain3/1
  in/1 -> Switch/1
  Memory/1 -> Switch/3
  Gain3/1 -> out/1

== system INS/Data_Fusion/Translation_Filter/CF/Verticle_Filter/Correct/GPS_Correct/GPS_Correct/Error_Scaling ==
  error_in : Inport
  rtk_valid : Inport  Port=2
  GPS_Error_Scaling : Subsystem
  RTK_Error_Scaling : Subsystem
  Switch : Switch  Criteria=u2 > Threshold
  error_out : Outport  VectorParamsAs1DForOutWhenUnconnected=off
  wires:
  error_in/1 -> RTK_Error_Scaling/1(error_in), GPS_Error_Scaling/1(error_in)
  rtk_valid/1 -> Switch/2
  RTK_Error_Scaling/1(error_out) -> Switch/1
  GPS_Error_Scaling/1(error_out) -> Switch/3
  Switch/1 -> error_out/1
